simulink model "DCmotor_maxon_Pcontrol"  (R2022b)
settings: Solver=VariableStepAuto  StartTime=0.0  StopTime=20  RelTol=1e-3
undefined symbols (not defined in the file): BM, eQ_s, Jgb, JM, KeM, KmM, Kp, LM, N, RM, sigbuilder_block, Ts
settings Model: Creator=riccardo  LastModifiedBy=Manu
settings SolverCC: AlgebraicLoopSolver=TrustRegion
settings DebuggingCC: UnconnectedInputMsg=warning  UnconnectedOutputMsg=warning  UnconnectedLineMsg=warning  SFMachineParentedDataDiag=warning
settings ModelReferenceCC: EnableRefExpFcnMdlSchedulingChecks=on
settings RTWCC: DLArmComputeVersion=19.05

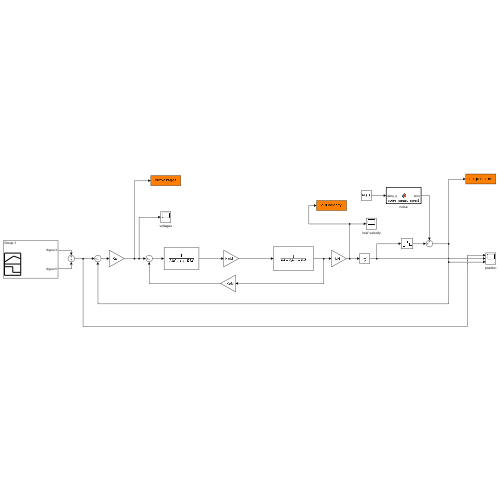
[thumbnail: Simulink's stored preview of the top-level diagram]
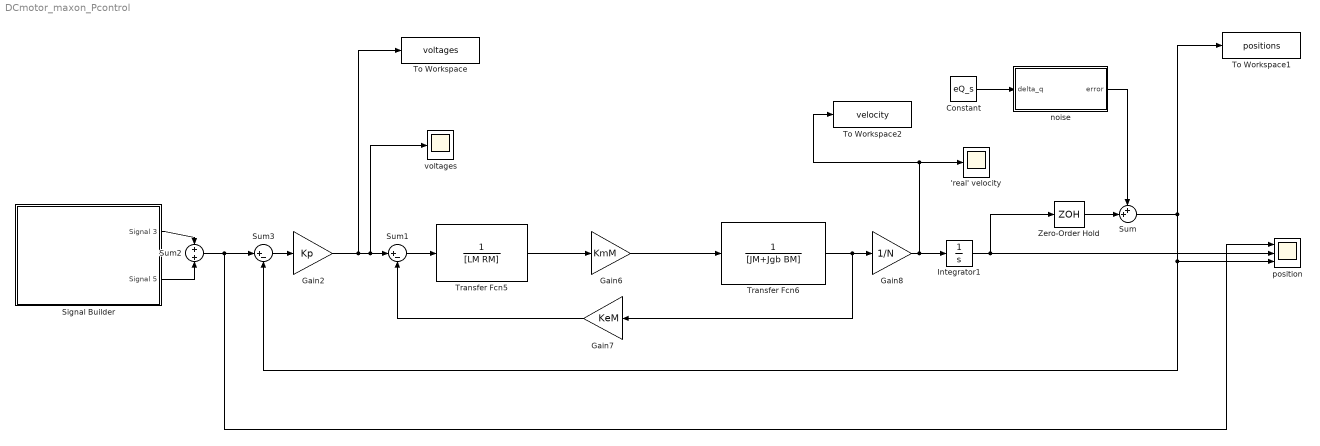
== system DCmotor_maxon_Pcontrol ==
  'real' velocity : Scope
  Constant : Constant  Value=eQ_s
  Gain2 : Gain  Gain=Kp
  Gain6 : Gain  Gain=KmM
  Gain7 : Gain  Gain=KeM
  Gain8 : Gain  Gain=1/N
  Integrator1 : Integrator
  Signal Builder : Subsystem  Tag=STV Subsys  LoadFcn=sigbuilder_block('load');  StartFcn=sigbuilder_block('start');  StopFcn=sigbuilder_block('stop');  ClipboardFcn=sigbuilder_block('clipboard');  mask(Sigbuilder block){tuvar=[0:10]}
      mask help: Simulink:masks:SigbuilderBlock_MD
      mask init:
      | if ~strcmp(get_param(bdroot(gcbh),'SimulationStatus'),'stopped') tuvar = sigbuilder_block('maskInit'); end
      settings: CopyFcn=sigbuilder_block('copy');  DeleteFcn=sigbuilder_block('delete');  ModelCloseFcn=sigbuilder_block('modelClose');  PreSaveFcn=sigbuilder_block('preSave');  PauseFcn=sigbuilder_block('pause');  ContinueFcn=sigbuilder_block('continue');  NameChangeFcn=sigbuilder_block('namechange');  OpenFcn=sigbuilder_block('open',[801.75 51.75 558 394.5 ]);  CloseFcn=sigbuilder_block('close');
      mask Display: plot(0, 0, 100, 100,[2, 2, 32, 32, 2], [68, 8, 8, 68, 68],[32, 2], [38, 38], [32, 19, 2],[53, 60, 44], [32, 17, 17, 2],[16, 16, 31, 31]);txt = getActiveGroup(gcbh);text(2, 100, txt,'verticalAlignment', 'top');
  Sum : Sum  Inputs=++|
  Sum1 : Sum  Inputs=|+-
  Sum2 : Sum
  Sum3 : Sum  Inputs=|+-
  To Workspace : ToWorkspace  VariableName=voltages  SaveFormat=Timeseries  SampleTime=Ts
  To Workspace1 : ToWorkspace  VariableName=positions  SaveFormat=Timeseries  SampleTime=Ts
  To Workspace2 : ToWorkspace  VariableName=velocity  SaveFormat=Timeseries  SampleTime=Ts
  Transfer Fcn5 : TransferFcn  Denominator=[LM RM]
  Transfer Fcn6 : TransferFcn  Denominator=[JM+Jgb BM]
  Zero-Order Hold : ZeroOrderHold  SampleTime=Ts
  noise : MATLAB Function  TreatAsAtomicUnit=on
  position : Scope  NumInputPorts=3
  voltages : Scope
  wires:
  Sum1/1 -> Transfer Fcn5/1
  Transfer Fcn5/1 -> Gain6/1
  Gain7/1 -> Sum1/2
  Transfer Fcn6/1 -> Gain7/1, Gain8/1
  Gain8/1 -> To Workspace2/1, 'real' velocity/1, Integrator1/1
  Integrator1/1 -> Zero-Order Hold/1, position/2
  Gain6/1 -> Transfer Fcn6/1
  Gain2/1 -> To Workspace/1, voltages/1, Sum1/1
  noise/1(error) -> Sum/1
  Constant/1 -> noise/1(delta_q)
  Zero-Order Hold/1 -> Sum/2
  Sum/1 -> To Workspace1/1, Sum3/2, position/3
  Sum2/1 -> position/1, Sum3/1
  Sum3/1 -> Gain2/1
  Signal Builder/1(Signal 3) -> Sum2/1
  Signal Builder/2(Signal 5) -> Sum2/2

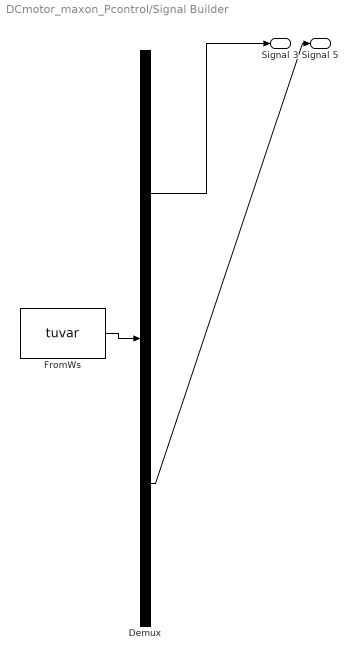
== system DCmotor_maxon_Pcontrol/Signal Builder ==
  Demux : Demux  Tag=STV Demux  Outputs=2
      settings: DisplayOption=none
  FromWs : FromWorkspace  Tag=STV FromWs  VariableName=tuvar
      SigBuilderData=|
      | common.afterFinalStr = 'Extrapolate'
      | common.sampleTime = 0
      | dataSet.timeRange = [0 25]
      | dataSet.name = 'Group 1'
      | sbobj.Groups.Name = 'Group 1'
      | sbobj.Groups.Signals(1).Name = 'Signal 3'
      | sbobj.Groups.Signals(1).XData = [0 1 1 2 2 5 5 8 8 9 9 10 10 11 11 15 15 18 18 19 19 21 21 22 22 23 23 25]
      | sbobj.Groups.Signals(1).YData = [1 1 -1 -1 1 1 -1 -1 1 1 -1 -1 1 1 -1 -1 1 1 -1 -1 1 1 -1 -1 1 1 -1 -1]
      | sbobj.Groups.Signals(2).Name = 'Signal 5'
      | sbobj.Groups.Signals(2).XData = [0 1 1 6 6 9 9 12 12 13 13 16 16 19 19 20 20 21 21 22 22 23 23 24 24 25]
      | sbobj.Groups.Signals(2).YData = [0.5 0.5 -0.5 -0.5 0.5 0.5 -0.5 -0.5 0.5 0.5 -0.5 -0.5 0.5 0.5 -0.5 -0.5 0.5 0.5 -0.5 -0.5 0.5 0.5 -0.5 -0.5 0.5 0.5]
      | sbobj.Groups.TimeRange = [0 25]
  Signal 3 : Outport  Tag=STV Outport
  Signal 5 : Outport  Tag=STV Outport  Port=2
  wires:
  FromWs/1 -> Demux/1
  Demux/1 -> Signal 3/1
  Demux/2 -> Signal 5/1

== matlab function DCmotor_maxon_Pcontrol/noise ==
  data: delta_q input; error output
function error = noise_measurement(delta_q)
if randn(1)>0
   error = delta_q;
else
    error = -delta_q;
end
